simulink model "wahadlo2"  (R2017b)
settings: Solver=ode4  StartTime=0.0  StopTime=100.0  FixedStep=0.01  RelTol=1e-3
settings Model: Creator=ba39216  LastModifiedBy=ba39216

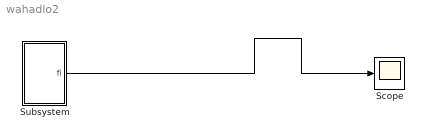
== system wahadlo2 ==
  Scope : Scope
  Subsystem : Subsystem  mask{m=10, k=1, l=3, g=10, fi0=90}
      mask prompts: m "masa"; k "tlumienie"; l "dlugosc"; g "przyspieszenie"; fi0 "kat_poczatkowy"
  wires:
  Subsystem/1(fi) -> Scope/1

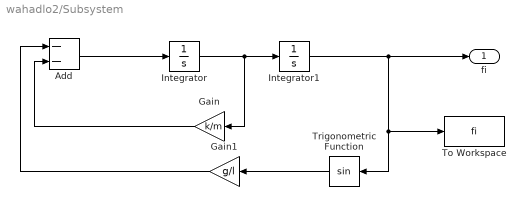
== system wahadlo2/Subsystem ==
  Add : Sum  Inputs=--
  Gain : Gain  Gain=k/m
  Gain1 : Gain  Gain=g/l
  Integrator : Integrator
  Integrator1 : Integrator  InitialCondition=fi0*pi/180
  To Workspace : ToWorkspace  VariableName=fi  SampleTime=-1
  Trigonometric Function : Trigonometry
  fi : Outport
  wires:
  Add/1 -> Integrator/1
  Trigonometric Function/1 -> Gain1/1
  Integrator/1 -> Gain/1, Integrator1/1
  Gain/1 -> Add/2
  Integrator1/1 -> fi/1, To Workspace/1, Trigonometric Function/1
  Gain1/1 -> Add/1
